simulink model "Simimplement152"  (R2021b)
settings: Solver=VariableStepAuto  StartTime=0.0  StopTime=10.0  RelTol=1e-3
values from neighbouring files (symbols this model uses):
  A152 = [-(L_Alpha/(U_0*m)) U_0 0; (L_Alpha*l_Alpha)/(U_0*I_y) 0  0;  0 1 0]    [Simulinkimplement152.m]
  B152 = [(T_c/m); ((l_c*T_c)/I_y); 0]    [Simulinkimplement152.m]
  C152 = eye(3,3)    [Simulinkimplement152.m]
  D152 = zeros(3,1)    [Simulinkimplement152.m]
  K_A = 6    [Simulinkimplement.m]    (also in Simulinkimplement152.m = 6.8; Simulinkimplement72.m = 52)
  K_c = 15    [Simulinkimplement.m]    (also in Simulinkimplement152.m; Simulinkimplement72.m)
  K_R = 0.5    [Simulinkimplement.m]    (also in Simulinkimplement152.m; Simulinkimplement72.m; Task1.m = 0.3; Task1time152sec.m = 0.3)
  theta_c = theta_c_deg*pi/180    (= 0.0872664625997)    [Simulinkimplement.m]    (also in Simulinkimplement152.m; Simulinkimplement72.m)
settings Model: Creator=raghu  LastModifiedBy=raghu
settings SolverCC: AlgebraicLoopSolver=TrustRegion
settings DebuggingCC: SFMachineParentedDataDiag=warning

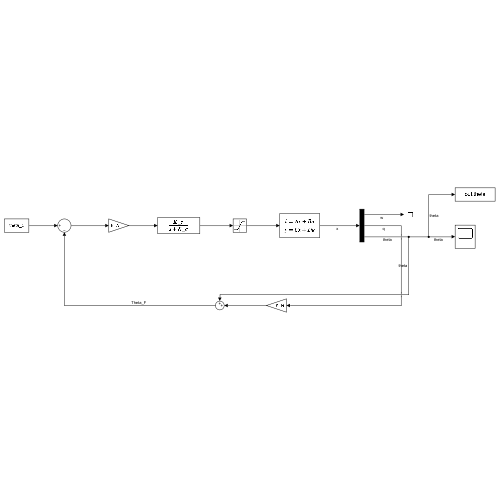
[thumbnail: Simulink's stored preview of the top-level diagram]
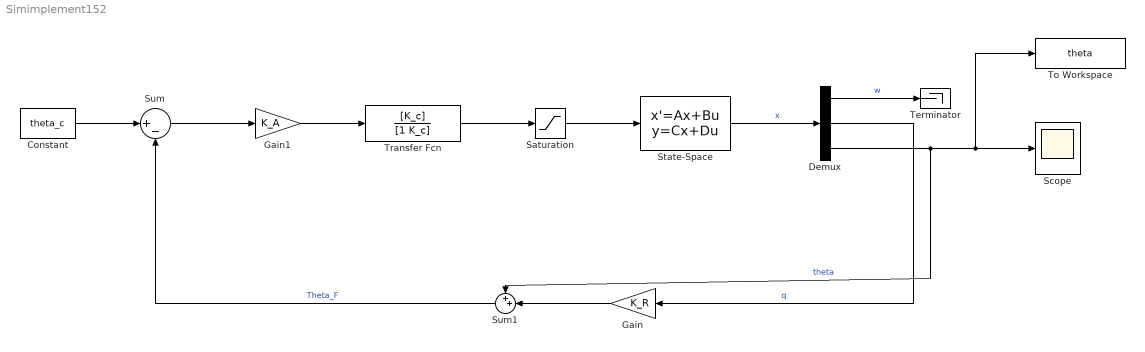
== system Simimplement152 ==
  Constant : Constant  Value=theta_c
  Demux : Demux  Outputs=3
  Gain : Gain  Gain=K_R
  Gain1 : Gain  Gain=K_A
  Saturation : Saturate
  Scope : Scope
  State-Space : StateSpace  A=A152  B=B152  C=C152  D=D152  InitialCondition=0
  Sum : Sum  Inputs=|+-
  Sum1 : Sum  Inputs=++|
  Terminator : Terminator
  To Workspace : ToWorkspace  VariableName=theta  SaveFormat=Timeseries  SampleTime=-1
  Transfer Fcn : TransferFcn  Numerator=[K_c]  Denominator=[1 K_c]
  wires:
  Gain1/1 -> Transfer Fcn/1
  Demux/2 -> Gain/1  "q"
  State-Space/1 -> Demux/1  "x"
  Demux/1 -> Terminator/1  "w"
  Sum/1 -> Gain1/1
  Sum1/1 -> Sum/2  "Theta_F"
  Transfer Fcn/1 -> Saturation/1
  Demux/3 -> Sum1/1, To Workspace/1, Scope/1  "theta"
  Constant/1 -> Sum/1
  Gain/1 -> Sum1/2
  Saturation/1 -> State-Space/1
